simulink model "BiquadPaparazzi"  (R2016b)
settings: Solver=VariableStepAuto  StartTime=0.0  StopTime=10.0  RelTol=1e-3
undefined symbols (not defined in the file or in its folder): pars
settings Model: Creator=kkajak  LastModifiedBy=Karl

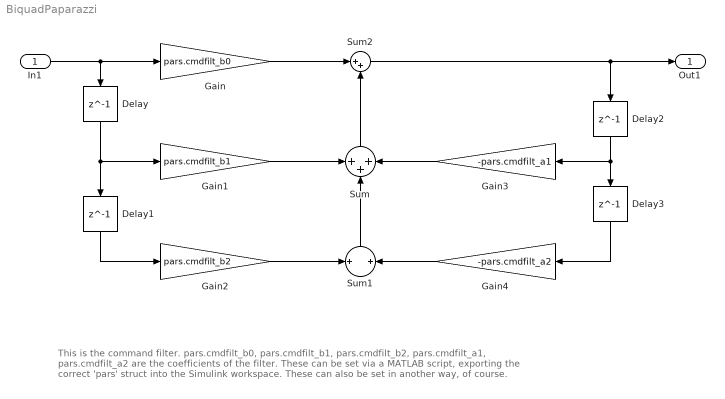
== system BiquadPaparazzi ==
  note: This is the command filter. pars.cmdfilt_b0, pars.cmdfilt_b1, pars.cmdfilt_b2, pars.cmdfilt_a1, pars.cmdfilt_a2 are the coefficients of the filter. These can be set via a MATLAB script,
      | exporting the correct 'pars' struct into the Simulink workspace. These can also be set in another way, of course.
  In1 : Inport  SampleTime=1/512
  Delay{,1..3} (4 alike) : Delay  DelayLength=1  InitialCondition=0
  Gain : Gain  Gain=pars.cmdfilt_b0
  Gain1 : Gain  Gain=pars.cmdfilt_b1
  Gain2 : Gain  Gain=pars.cmdfilt_b2
  Gain3 : Gain  Gain=-pars.cmdfilt_a1
  Gain4 : Gain  Gain=-pars.cmdfilt_a2
  Sum : Sum  Inputs=+++
  Sum1 : Sum  Inputs=+||+
  Sum2 : Sum  Inputs=|++
  Out1 : Outport
  wires:
  Gain/1 -> Sum2/1
  In1/1 -> Delay/1, Gain/1
  Gain1/1 -> Sum/1
  Gain2/1 -> Sum1/1
  Delay/1 -> Delay1/1, Gain1/1
  Delay1/1 -> Gain2/1
  Gain3/1 -> Sum/3
  Gain4/1 -> Sum1/2
  Delay2/1 -> Delay3/1, Gain3/1
  Delay3/1 -> Gain4/1
  Sum/1 -> Sum2/2
  Sum1/1 -> Sum/2
  Sum2/1 -> Delay2/1, Out1/1
